simulink model "ClarkTransformationMatrix"  (R2022a)
settings: Solver=VariableStepAuto  StartTime=0.0  StopTime=10.0  RelTol=1e-3
settings Model: Creator=jff_1  LastModifiedBy=jff_1

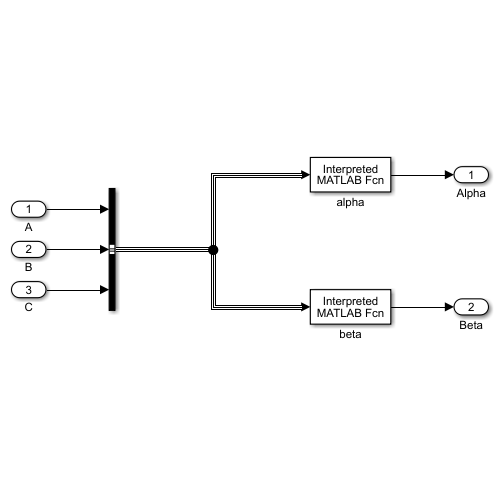
[thumbnail: Simulink's stored preview of the top-level diagram]
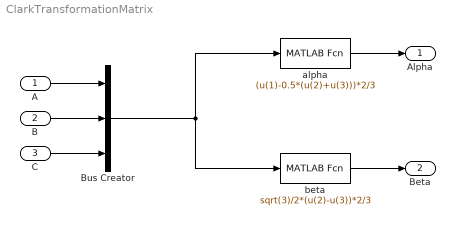
== system ClarkTransformationMatrix ==
  A : Inport
  B : Inport  Port=2
  C : Inport  Port=3
  Bus Creator : BusCreator  Inputs=3
  alpha : MATLABFcn  MATLABFcn=(u(1)-0.5*(u(2)+u(3)))*2/3
  beta : MATLABFcn  MATLABFcn=sqrt(3)/2*(u(2)-u(3))*2/3
  Alpha : Outport
  Beta : Outport  Port=2
  wires:
  A/1 -> Bus Creator/1
  B/1 -> Bus Creator/2
  C/1 -> Bus Creator/3
  Bus Creator/1 -> beta/1, alpha/1
  alpha/1 -> Alpha/1
  beta/1 -> Beta/1
